simulink model "DuckCarSimORIGINAL"  (R2023b)
settings: Solver=VariableStepAuto  StartTime=0.0  StopTime=10  MaxStep=0.05  RelTol=1e-3  EnableMultiTasking=on
values from neighbouring files (symbols this model uses):
  b = chosenIndecies(itt)    [DuckCarLab3.m]
undefined symbols (not defined in the file or in its folder): Km, m, tau
settings Model: Creator=AllisonBT  LastModifiedBy=n8dsa
settings SolverCC: AlgebraicLoopSolver=TrustRegion
settings DataIOCC: ReturnWorkspaceOutputs=off
settings OptimizationCC: LifeSpan=inf
settings DebuggingCC: UnconnectedInputMsg=warning  UnconnectedOutputMsg=warning  UnconnectedLineMsg=warning  SFUnexpectedBacktrackingDiag=warning  SFNoUnconditionalDefaultTransitionDiag=warning  ArithmeticOperatorsInVariantConditions=warning
settings ModelReferenceCC: EnableRefExpFcnMdlSchedulingChecks=on
settings SFSimCC: SimUseLocalCustomCode=off  CustomCodeUndefinedFunction=UseInterfaceOnly
settings RTWCC: RTWUseLocalCustomCode=off
settings CodeAppCC: StateflowObjectComments=on
settings GRTTargetCC: TargetLangStandard=C89/C90 (ANSI)
settings ConfigComp: CovMetricSettings=dw  CovSaveCumulativeToWorkspaceVar=on  CovSaveSingleToWorkspaceVar=on  CovExternalEMLEnable=off

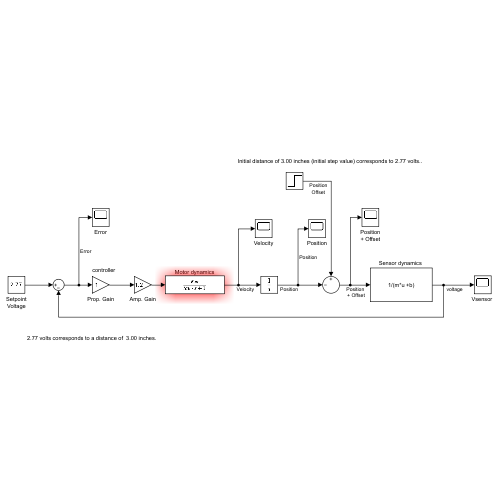
[thumbnail: Simulink's stored preview of the top-level diagram]
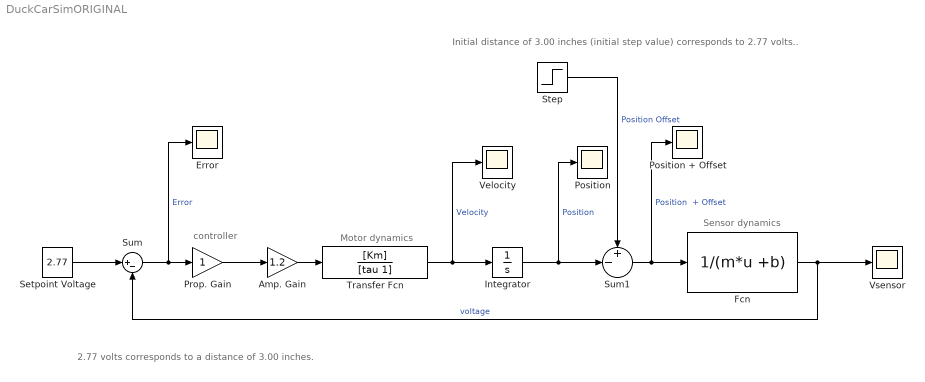
== system DuckCarSimORIGINAL ==
  note: Sensor dynamics
  note: Motor dynamics
  note: 2.77 volts corresponds to a distance of 3.00 inches.
  note: Initial distance of 3.00 inches (initial step value) corresponds to 2.77 volts..
  note: controller
  Amp. Gain : Gain  Gain=1.2
  Error : Scope
  Fcn : Fcn  Expr=1/(m*u +b)
  Integrator : Integrator
  Position : Scope
  Position + Offset : Scope
  Prop. Gain : Gain
  Setpoint Voltage : Constant  Value=2.77
  Step : Step  Before=3  After=6  SampleTime=0
  Sum : Sum  Inputs=|+-
  Sum1 : Sum  Inputs=+-|
  Transfer Fcn : TransferFcn  Numerator=[Km]  Denominator=[tau 1]
  Velocity : Scope
  "Vsensor " : Scope
  wires:
  Amp. Gain/1 -> Transfer Fcn/1
  Prop. Gain/1 -> Amp. Gain/1
  Sum/1 -> Error/1, Prop. Gain/1  "Error"
  Fcn/1 -> "Vsensor "/1, Sum/2  "voltage"
  Setpoint Voltage/1 -> Sum/1
  Transfer Fcn/1 -> Velocity/1, Integrator/1  "Velocity"
  Step/1 -> Sum1/1  "Position Offset"
  Sum1/1 -> Position + Offset/1, Fcn/1  "Position  + Offset"
  Integrator/1 -> Position/1, Sum1/2  "Position"
